simulink model "b_Trabajo_final_FSK"  (R2023b)
settings: Solver=FixedStepDiscrete  StartTime=0.0  StopTime=503983  RelTol=1e-3
libraries: commdigbbndfm2 x2, commchan3 x1, commsink2 x1
settings Model: Creator=Enmanel Toribio  LastModifiedBy=Enmanel Toribio

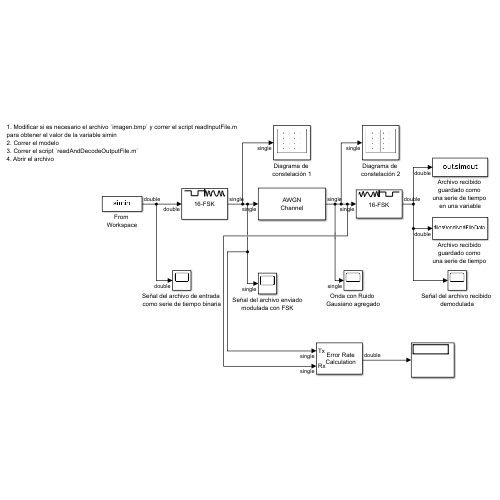
[thumbnail: Simulink's stored preview of the top-level diagram]
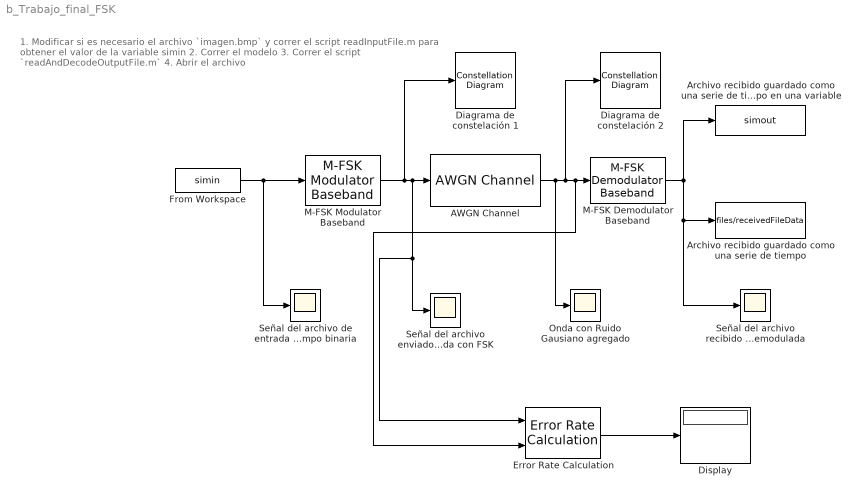
== system b_Trabajo_final_FSK ==
  note: 1. Modificar si es necesario el archivo `imagen.bmp` y correr el script readInputFile.m para obtener el valor de la variable simin
      | 2. Correr el modelo
      | 3. Correr el script `readAndDecodeOutputFile.m`
      | 4. Abrir el archivo
  AWGN Channel : commchan3/AWGN Channel  LegacyMode=off  NoiseMethod="Signal to noise ratio  (SNR)"  noiseMode="Signal to noise ratio  (SNR)"  EbNo=10  EsNo=10  SNR=20  BitsPerSymbol=1  SignalPower=1  SamplesPerSymbol=1  SymbolPeriod=1  VarianceSource=Parameter  Variance=1  RandomStream=Global stream  Seed=67  SimulateUsing=Code generation
  "Archivo recibido guardado como una serie de tiempo " : ToFile  Filename=files/receivedFileData  MatrixName=received_binary_data  SampleTime=1
  Archivo recibido guardado como una serie de tiempo en una variable : ToWorkspace  VariableName=simout  SaveFormat=Timeseries  SampleTime=1
  Diagrama de constelación 1 : ConstellationDiagram  WindowPosition=[577.000000,131.000000,600.000000,521.000000,]  Visible=on  ScopeFrameLocation=window  DefaultConfigurationName=comm.scopes.ConstellationDiagramBlockCfg
  Diagrama de constelación 2 : ConstellationDiagram  WindowPosition=[1242.000000,199.000000,600.000000,600.000000,]  Visible=on  ScopeFrameLocation=window  DefaultConfigurationName=comm.scopes.ConstellationDiagramBlockCfg
  Display : Display
  Error Rate Calculation : commsink2/Error Rate Calculation  N=0  st_delay=0  cp_mode=Entire frame  subframe=[]  PMode=Port  WsName=ErrorVec  RsMode2=off  stop=off  numErr=100  maxBits=1e6
      settings: LibrarySourceBlock=|
      | commhdlsink/Error Rate
      | Calculation
  From Workspace : FromWorkspace  VariableName=simin  SampleTime=1
  M-FSK Demodulator Baseband : commdigbbndfm2/M-FSK Demodulator Baseband  M=16  OutType=Integer  Dec=Gray  freqSep=100  numSamp=8  RateOptions=Enforce single-rate processing  outDataType=double
  M-FSK Modulator Baseband : commdigbbndfm2/M-FSK Modulator Baseband  M=16  InType=Integer  Enc=Gray  freqSep=100  phaseType=Continuous  numSamp=8  RateOptions=Enforce single-rate processing  outDataType=single
  Onda con Ruido Gausiano agregado : Scope
  Señal del archivo de entrada como serie de tiempo binaria : Scope
  Señal del archivo enviado modulada con FSK : Scope
  Señal del archivo recibido demodulada : Scope
  wires:
  From Workspace/1 -> Señal del archivo de entrada como serie de tiempo binaria/1, M-FSK Modulator Baseband/1
  M-FSK Demodulator Baseband/1 -> "Archivo recibido guardado como una serie de tiempo "/1, Señal del archivo recibido demodulada/1, Archivo recibido guardado como una serie de tiempo en una variable/1
  M-FSK Modulator Baseband/1 -> Diagrama de constelación 1/1, Error Rate Calculation/1, Señal del archivo enviado modulada con FSK/1, AWGN Channel/1
  Error Rate Calculation/1 -> Display/1
  AWGN Channel/1 -> Onda con Ruido Gausiano agregado/1, Diagrama de constelación 2/1, Error Rate Calculation/2, M-FSK Demodulator Baseband/1
